simulink model "single_phase_hw_dlr"  (Simulink 6.1)
settings: Solver=ode23tb  StartTime=0.0  StopTime=0.29999  MaxStep=1e-4  RelTol=1e-3  AbsTol=.01
libraries: powerlib x7
settings Model: LastModifiedBy=ThinkPad
settings DebuggingCC: SolverPrmCheckMsg=warning

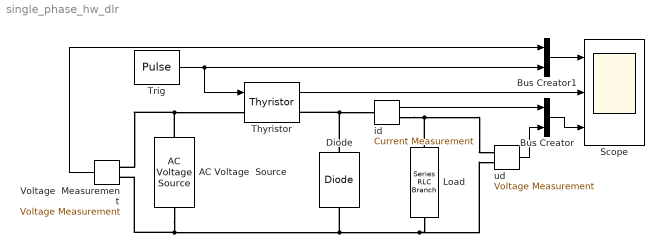
== system single_phase_hw_dlr ==
  AC Voltage  Source : powerlib/Electrical Sources/AC Voltage Source  Orientation=up  Amplitude=100  Phase=0  Frequency=50  SampleTime=0  Measurements=None
  Bus Creator : BusCreator  DialogController=Simulink.DDGSource_Bus  Inputs=2
  Bus Creator1 : BusCreator  DialogController=Simulink.DDGSource_Bus  Inputs=2
  Diode : powerlib/Power Electronics/Diode  Orientation=up  Ron=0.01  Lon=0  Vf=0.8  IC=0  Rs=500  Cs=250e-9  Measurements=off
  Load : powerlib/Elements/Series RLC Branch  Orientation=down  PhysicalDomain=powersysdomain  SubClassName=unknown  LeftPortType=p1  RightPortType=p1  LConnTagsString=__new0  RConnTagsString=__new0  Resistance=1  Inductance=0.1  Capacitance=inf  Measurements=None
  Scope : Scope  NumInputPorts=3
      settings: TimeRange=0.1  YMin=-100~-100~0  YMax=100~100~100  Decimation=5  SampleInput=on  SampleTime=1e-4
  Thyristor : powerlib/Power Electronics/Thyristor  Ron=0.01  Lon=0  Vf=0.8  IC=0  Rs=1000  Cs=100e-9  Measurements=on
  Trig : DiscretePulseGenerator  PulseType=Time based  Amplitude=10  Period=0.02  PulseWidth=5  PhaseDelay=0.0025
  Voltage  Measurement : powerlib/Measurements/Voltage Measurement  Orientation=left  PhasorSimulation=off  OutputType=Complex  PSBequivalent=0
  id : powerlib/Measurements/Current Measurement  PhasorSimulation=off  OutputType=Complex  PSBequivalent=0
  ud : powerlib/Measurements/Voltage Measurement  PhasorSimulation=off  OutputType=Complex  PSBequivalent=0
  wires:
  Trig/1 -> Thyristor/1, Bus Creator1/2
  Thyristor/1 -> Scope/2
  ud/1 -> Bus Creator/2
  Bus Creator/1 -> Scope/3
  id/1 -> Bus Creator/1
  Bus Creator1/1 -> Scope/1
  Voltage  Measurement/1 -> Bus Creator1/1
  connections:
  AC Voltage  Source/RConn1 -- Thyristor/LConn1 -- Voltage  Measurement/LConn1
  Load/LConn1 -- ud/LConn1 -- id/RConn1
  AC Voltage  Source/LConn1 -- ud/LConn2 -- Load/RConn1 -- Diode/LConn1 -- Voltage  Measurement/LConn2
  Diode/RConn1 -- Thyristor/RConn1 -- id/LConn1
